simulink model "observerModel_GVS"  (R2024a)
settings: Solver=ode15s  StartTime=0.0  StopTime=duration  MaxStep=0.02  RelTol=0.02  AbsTol=0.02  EnableMultiTasking=on
values from neighbouring files (symbols this model uses):
  delta_t = time(2) - time (1)    [Observer_Analysis.m]
  f_oto = 2    [Observer_Analysis.m]
  f_scc = 2    [Observer_Analysis.m]
  GG0 = [0 0 -hypo]'    [Observer_Analysis.m]
  IrregDepol = tf(num,den)    [Observer_Analysis.m]
  IrregHyperpol = tf(num,den)    [Observer_Analysis.m]
  IrregSCC2Physical = inv(IrregSCCnf)    [Observer_Analysis.m]
  kaa = -4*[1 1 1]'    [Observer_Analysis.m]
  kfg = 4*[1 1 1]'    [Observer_Analysis.m]
  kfw = 8*[1 1 1]'    [Observer_Analysis.m]
  KGVS = s2(1)*pi/180    [Observer_Analysis.m]
  KLeft = 1-KRight    (= 0.5)    [Observer_Analysis.m]
  KReg = s2(2)    [Observer_Analysis.m]
  KRight = 0.5    [Observer_Analysis.m]
  kwg = 1*[1 1 1]'    [Observer_Analysis.m]
  kww = 8*[1 1 1]'    [Observer_Analysis.m]
  oto_a = 60*[1 1 1]'    [Observer_Analysis.m]
  oto_Ka = 1.3*[1 1 1]'    [Observer_Analysis.m]
  Q0 = [cos(E_angle/2) E(1)*sin(E_angle/2) E(2)*sin(E_angle/2) E(3)*sin(E_angle/2)]'    [Observer_Analysis.m]
  RegDepol = tf(num,den)    [Observer_Analysis.m]
  RegHyperpol = tf(num,den)    [Observer_Analysis.m]
  RegSCC2Physical = inv(RegSCCnf)    [Observer_Analysis.m]
  tau_a = tau_a_value*[1 1 1]'    [Observer_Analysis.m]
  tau_scc = tau_scc_value*[1 1 1]'    [Observer_Analysis.m]
(part 1 of 2)
settings Model: Creator=Newman  LastModifiedBy=caroa
settings SolverCC: AutoScaleAbsTol=off  AlgebraicLoopSolver=TrustRegion
settings DataIOCC: SaveFormat=Array  SignalLoggingSaveFormat=ModelDataLogs  SaveOutput=off  SaveTime=off  ReturnWorkspaceOutputs=off
settings OptimizationCC: ReuseModelBlockBuffer=off  ExpressionDepthLimit=2147483647  InitFltsAndDblsToZero=on  LifeSpan=inf
settings DebuggingCC: SaveWithParameterizedLinksMsg=none  UnderspecifiedInitializationDetection=Classic  MergeDetectMultiDrivingBlocksExec=none  SolverPrmCheckMsg=warning  FcnCallInpInsideContextMsg=warning  UnconnectedInputMsg=warning  UnconnectedOutputMsg=warning  UnconnectedLineMsg=warning  StateNameClashWarn=warning  SFUnexpectedBacktrackingDiag=warning  SFNoUnconditionalDefaultTransitionDiag=warning  SFExecutionAtInitializationDiag=none  ArithmeticOperatorsInVariantConditions=warning
settings HardwareCC: ProdBitPerPointer=32  ProdBitPerSizeT=32  ProdBitPerPtrDiffT=32  ProdLargestAtomicFloat=None  ProdIntDivRoundTo=Undefined  ProdEndianess=Unspecified  ProdWordSize=32  ProdHWDeviceType=32-bit Generic
settings ModelReferenceCC: EnableRefExpFcnMdlSchedulingChecks=on  PropagateSignalLabelsOutOfModel=off
settings SFSimCC: SimUseLocalCustomCode=off  CustomCodeUndefinedFunction=UseInterfaceOnly
settings RTWCC: RTWUseLocalCustomCode=off  GPUComputeCapability=3.5  DLArmComputeVersion=19.05
settings CodeAppCC: StateflowObjectComments=on
settings GRTTargetCC: TargetFcnLib=ansi_tfl_tmw.mat  TargetLangStandard=C89/C90 (ANSI)  CombineOutputUpdateFcns=off  GRTInterface=on
settings ConfigComp: CovMetricSettings=dw  CovSaveCumulativeToWorkspaceVar=on  CovSaveSingleToWorkspaceVar=on  CovExternalEMLEnable=off

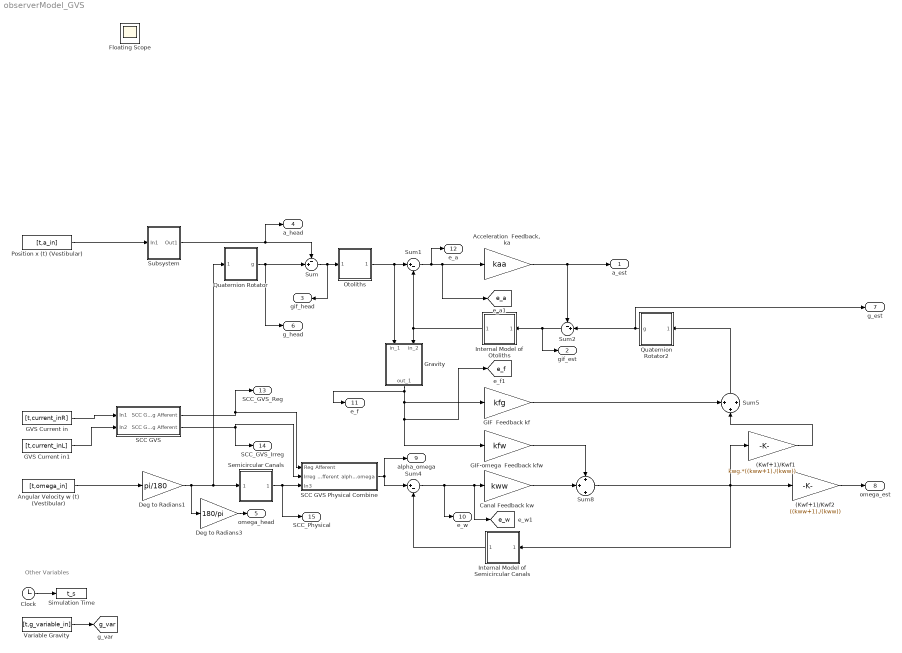
== system observerModel_GVS ==
  note: Other Variables
  (Kwf+1)/Kwf1 : Gain  Gain=kwg.*((kww+1)./(kww))  SaturateOnIntegerOverflow=on  OutDataTypeStr=Inherit: Same as input  ParamDataTypeStr=Inherit: Same as input
  (Kwf+1)/Kwf2 : Gain  Gain=((kww+1)./(kww))  SaturateOnIntegerOverflow=on  OutDataTypeStr=Inherit: Same as input  ParamDataTypeStr=Inherit: Same as input
  "Acceleration  Feedback, ka" : Gain  Gain=kaa  SaturateOnIntegerOverflow=on  OutDataTypeStr=Inherit: Same as input  ParamDataTypeStr=Inherit: Same as input
  Angular Velocity w (t) (Vestibular) : FromWorkspace  VariableName=[t,omega_in]  ZeroCross=off
  Canal Feedback kw : Gain  Gain=kww  SaturateOnIntegerOverflow=on  OutDataTypeStr=Inherit: Same as input  ParamDataTypeStr=Inherit: Same as input
  Clock : Clock
  Deg to Radians1 : Gain  Gain=pi/180  SaturateOnIntegerOverflow=on  OutDataTypeStr=Inherit: Same as input  ParamDataTypeStr=Inherit: Same as input
  Deg to Radians3 : Gain  Gain=180/pi  SaturateOnIntegerOverflow=on  OutDataTypeStr=Inherit: Same as input  ParamDataTypeStr=Inherit: Same as input
  GIF  Feedback kf : Gain  Gain=kfg  SaturateOnIntegerOverflow=on  OutDataTypeStr=Inherit: Same as input  ParamDataTypeStr=Inherit: Same as input
  GIF-omega  Feedback kfw : Gain  Gain=kfw  SaturateOnIntegerOverflow=on  OutDataTypeStr=Inherit: Same as input  ParamDataTypeStr=Inherit: Same as input
  GVS Current in : FromWorkspace  VariableName=[t,current_inR]  ZeroCross=off
  GVS Current in1 : FromWorkspace  VariableName=[t,current_inL]  ZeroCross=off
  Gravity : Subsystem
  Internal Model of Otoliths : Subsystem
      mask Display: fprintf('<OTO>')
  Internal Model of Semicircular Canals : Subsystem
      mask Display: fprintf('<SCC>')
  Otoliths : Subsystem
      mask Display: fprintf('OTO')
  Position x (t) (Vestibular) : FromWorkspace  VariableName=[t,a_in]  ZeroCross=off
  Quaternion Rotator : Subsystem
      mask Display: fprintf('G(w)')
  Quaternion Rotator2 : Subsystem
      mask Display: fprintf('Gest(w)')
  "SCC GVS " : Subsystem
  SCC GVS Physical Combine : Subsystem
  Semicircular Canals : Subsystem
      mask Display: fprintf('SCC')
  Simulation Time : ToWorkspace  VariableName=t_s
      settings: MaxDataPoints=100000
  Subsystem : Subsystem
      mask Display: fprintf('TH(w)')
  Sum : Sum  Inputs=-+|
  Sum1 : Sum  Inputs=|+-
  Sum2 : Sum  Inputs=-+|
  Sum4 : Sum  Inputs=|+-
  Sum5 : Sum  Inputs=+|+|+
  Sum8 : Sum  Inputs=+|+|+
  Variable Gravity : FromWorkspace  VariableName=[t,g_variable_in]  ZeroCross=off
  a_est : Outport
  gif_est : Outport  Port=2
  gif_head : Outport  Port=3
  a_head : Outport  Port=4
  omega_head : Outport  Port=5
  g_head : Outport  Port=6
  g_est : Outport  Port=7
  omega_est : Outport  Port=8
  alpha_omega : Outport  Port=9
  e_w : Outport  Port=10
  e_f : Outport  Port=11
  e_a : Outport  Port=12
  SCC_GVS_Reg : Outport  Port=13
  SCC_GVS_Irreg : Outport  Port=14
  SCC_Physical : Outport  Port=15
  Floating Scope : Scope
  tag scope: e_a=global, e_f=global, e_w=global, g_var=global
  wires:
  Clock/1 -> Simulation Time/1
  Quaternion Rotator/1(g) -> Sum/2, g_head/1
  Position x (t) (Vestibular)/1 -> Subsystem/1(In1)
  Sum/1 -> gif_head/1, Otoliths/1(Inport)
  Sum1/1 -> [e_a], "Acceleration  Feedback, ka"/1, e_a/1
  Otoliths/1(Outport) -> Sum1/1, Gravity/1(in_1)
  Sum2/1 -> gif_est/1, Internal Model of Otoliths/1(Inport)
  "Acceleration  Feedback, ka"/1 -> Sum2/1, a_est/1
  Gravity/1(out_1) -> GIF-omega  Feedback kfw/1, [e_f], GIF  Feedback kf/1, e_f/1
  GIF  Feedback kf/1 -> Sum5/1
  Sum5/1 -> Quaternion Rotator2/1(omega_rad_est)
  Sum4/1 -> [e_w], Canal Feedback kw/1, e_w/1
  GIF-omega  Feedback kfw/1 -> Sum8/1
  Canal Feedback kw/1 -> Sum8/2
  Internal Model of Semicircular Canals/1(Outport) -> Sum4/2
  Internal Model of Otoliths/1(Outport) -> Gravity/2(in_2), Sum1/2
  Sum8/1 -> (Kwf+1)/Kwf2/1, (Kwf+1)/Kwf1/1, Internal Model of Semicircular Canals/1(Inport)
  Quaternion Rotator2/1(g) -> g_est/1, Sum2/2
  Angular Velocity w (t) (Vestibular)/1 -> Deg to Radians1/1
  Deg to Radians3/1 -> omega_head/1
  Variable Gravity/1 -> [g_var]
  Deg to Radians1/1 -> Quaternion Rotator/1(omega_rad), Semicircular Canals/1(Inport), Deg to Radians3/1
  Subsystem/1(Out1) -> Sum/1, a_head/1
  (Kwf+1)/Kwf2/1 -> omega_est/1
  (Kwf+1)/Kwf1/1 -> Sum5/2
  GVS Current in/1 -> "SCC GVS "/1(In1)
  SCC GVS Physical Combine/1(alpha_omega) -> alpha_omega/1, Sum4/1
  "SCC GVS "/2(SCC GVS Irreg Afferent) -> SCC GVS Physical Combine/2(Irreg Afferent), SCC_GVS_Irreg/1
  "SCC GVS "/1(SCC GVS Reg Afferent) -> SCC_GVS_Reg/1, SCC GVS Physical Combine/1(Reg Afferent)
  Semicircular Canals/1(Outport) -> SCC_Physical/1, SCC GVS Physical Combine/3(In3)
  GVS Current in1/1 -> "SCC GVS "/2(In2)

== system observerModel_GVS/Gravity ==
  in_1 : Inport
  in_2 : Inport  Port=2
  Cross Product : Subsystem  mask(Nick's Library){}
      mask help: Cross Product
      mask Help: Cross Product
      mask Display: disp('--> -->\nu x v')
  Dot Product : DotProduct  OutDataTypeStr=Inherit: Inherit via internal rule
  Normalize : Subsystem
      mask Display: disp('->\nu\n__\n->\n|u|')
  Normalize1 : Subsystem
      mask Display: disp('->\nu\n__\n->\n|u|')
  Normalize2 : Subsystem
      mask Display: disp('->\nu\n__\n->\n|u|')
  Product : Product  InputSameDT=on  RndMeth=Zero  SaturateOnIntegerOverflow=on  OutDataTypeStr=Inherit: Same as first input
  Trigonometric Function : Trigonometry  Operator=acos
  out_1 : Outport  InitialOutput=0
  wires:
  Trigonometric Function/1 -> Product/2
  Product/1 -> out_1/1
  Normalize1/1(out_1) -> Dot Product/1
  Normalize/1(out_1) -> Dot Product/2
  in_1/1 -> Normalize1/1(in_1), Cross Product/1(in_1)
  Normalize2/1(out_1) -> Product/1
  Dot Product/1 -> Trigonometric Function/1
  Cross Product/1(out_1) -> Normalize2/1(in_1)
  in_2/1 -> Normalize/1(in_1), Cross Product/2(in_2)

== system observerModel_GVS/Internal Model of Otoliths ==
  note: Z otolith
  note: Y otolith
  note: X otolith
  Inport : Inport
  Demux : Demux  Outputs=3
      settings: DisplayOption=none
  Mux : Mux  Inputs=3
  Otolith : Subsystem
  Otolith1 : Subsystem
  Otolith2 : Subsystem
  Outport : Outport  InitialOutput=0
  wires:
  Otolith2/1(out_1) -> Mux/3
  Otolith/1(out_1) -> Mux/1
  Otolith1/1(out_1) -> Mux/2
  Demux/3 -> Otolith2/1(in_1)
  Demux/1 -> Otolith/1(in_1)
  Demux/2 -> Otolith1/1(in_1)
  Inport/1 -> Demux/1
  Mux/1 -> Outport/1

== system observerModel_GVS/Internal Model of Semicircular Canals ==
  note: Z canal
  note: Y canal
  note: X canal
  Inport : Inport
  Demux : Demux  Outputs=3
      settings: DisplayOption=none
  Mux : Mux  Inputs=3
  Zero-Pole : ZeroPole  Zeros=[0]  Poles=[-1/tau_scc(1);-2*pi*f_scc]  Gain=[(2*pi*f_scc)]
  Zero-Pole1 : ZeroPole  Zeros=[0]  Poles=[-1/tau_scc(2);-2*pi*f_scc]  Gain=[(2*pi*f_scc)]
  Zero-Pole2 : ZeroPole  Zeros=[0]  Poles=[-1/tau_scc(3);-2*pi*f_scc]  Gain=[(2*pi*f_scc)]
  Outport : Outport  InitialOutput=0
  wires:
  Inport/1 -> Demux/1
  Demux/3 -> Zero-Pole2/1
  Demux/1 -> Zero-Pole/1
  Demux/2 -> Zero-Pole1/1
  Zero-Pole2/1 -> Mux/3
  Zero-Pole1/1 -> Mux/2
  Zero-Pole/1 -> Mux/1
  Mux/1 -> Outport/1

== system observerModel_GVS/Otoliths ==
  Inport : Inport
  Demux : Demux  Outputs=3
      settings: DisplayOption=none
  Mux : Mux  Inputs=3
  X Graviceptor : Subsystem
  Y Graviceptor : Subsystem
  Z Graviceptor : Subsystem
  Outport : Outport  InitialOutput=0
  wires:
  Z Graviceptor/1(out_1) -> Mux/3
  X Graviceptor/1(out_1) -> Mux/1
  Y Graviceptor/1(out_1) -> Mux/2
  Demux/3 -> Z Graviceptor/1(in_1)
  Demux/1 -> X Graviceptor/1(in_1)
  Demux/2 -> Y Graviceptor/1(in_1)
  Inport/1 -> Demux/1
  Mux/1 -> Outport/1

== system observerModel_GVS/Quaternion Rotator ==
  omega_rad : Inport
  Head to Limbic Angular Velocity Transform : Subsystem
  Quaternion Integrator : Subsystem
  Quaternion to Direction Cosine : Subsystem
  Quaternion to Euler Angles : Subsystem
  Rotation : Subsystem
  SVV : ToWorkspace  VariableName=SVV  SampleTime=-1
  Tilt : ToWorkspace  VariableName=tilt  SampleTime=-1
  Tilt & SVV : Subsystem
  To Workspace : ToWorkspace  VariableName=azimuth_head  SampleTime=-1
  To Workspace2 : ToWorkspace  VariableName=euler_head  SampleTime=-1
  g : Outport
  tag scope: D_Cos=global, R_head=global
  wires:
  Quaternion Integrator/1(q) -> Quaternion to Direction Cosine/1(q), Quaternion to Euler Angles/1(q)
  Quaternion to Direction Cosine/1(D_Cos) -> Rotation/1(D_Cos), Head to Limbic Angular Velocity Transform/2(D_Cos), [D_Cos]
  omega_rad/1 -> Quaternion Integrator/1(omega_head), Rotation/2(omega_rad), Head to Limbic Angular Velocity Transform/1(omega_head)
  Rotation/1(g) -> g/1, Tilt & SVV/1(g)
  Rotation/2(azimuth) -> To Workspace/1
  Head to Limbic Angular Velocity Transform/1(R_limbic) -> [R_head]
  Quaternion to Euler Angles/1(Euler) -> To Workspace2/1
  Tilt & SVV/1(Tilt) -> Tilt/1
  Tilt & SVV/2(SVV) -> SVV/1

== system observerModel_GVS/Quaternion Rotator2 ==
  omega_rad_est : Inport
  Head to Limbic Angular Velocity Transform Rotation Matrix : Subsystem
  Quaternion Integrator : Subsystem
  Quaternion to Direction Cosine : Subsystem
  Quaternion to Euler Angles : Subsystem
  Rotation : Subsystem
  SVV Est : ToWorkspace  VariableName=SVV_est  SampleTime=-1
  Tilt & SVV : Subsystem
  Tilt Est : ToWorkspace  VariableName=tilt_est  SampleTime=-1
  To Workspace : ToWorkspace  VariableName=azimuth_est  SampleTime=-1
  To Workspace2 : ToWorkspace  VariableName=euler_est  SampleTime=-1
  g : Outport
  tag scope: D_Cos_est=global, R_est=global
  wires:
  Quaternion Integrator/1(q) -> Quaternion to Direction Cosine/1(q), Quaternion to Euler Angles/1(q)
  Quaternion to Direction Cosine/1(D_Cos) -> Rotation/1(D_Cos), [D_Cos_est], Head to Limbic Angular Velocity Transform Rotation Matrix/2(D_Cos)
  omega_rad_est/1 -> Quaternion Integrator/1(omega_rad_est), Rotation/2(omega_rad), Head to Limbic Angular Velocity Transform Rotation Matrix/1(omega_est)
  Rotation/1(g) -> g/1, Tilt & SVV/1(g)
  Rotation/2(azimuth) -> To Workspace/1
  Head to Limbic Angular Velocity Transform Rotation Matrix/1(R_limbic_est) -> [R_est]
  Quaternion to Euler Angles/1(Euler) -> To Workspace2/1
  Tilt & SVV/1(Tilt) -> Tilt Est/1
  Tilt & SVV/2(SVV) -> SVV Est/1

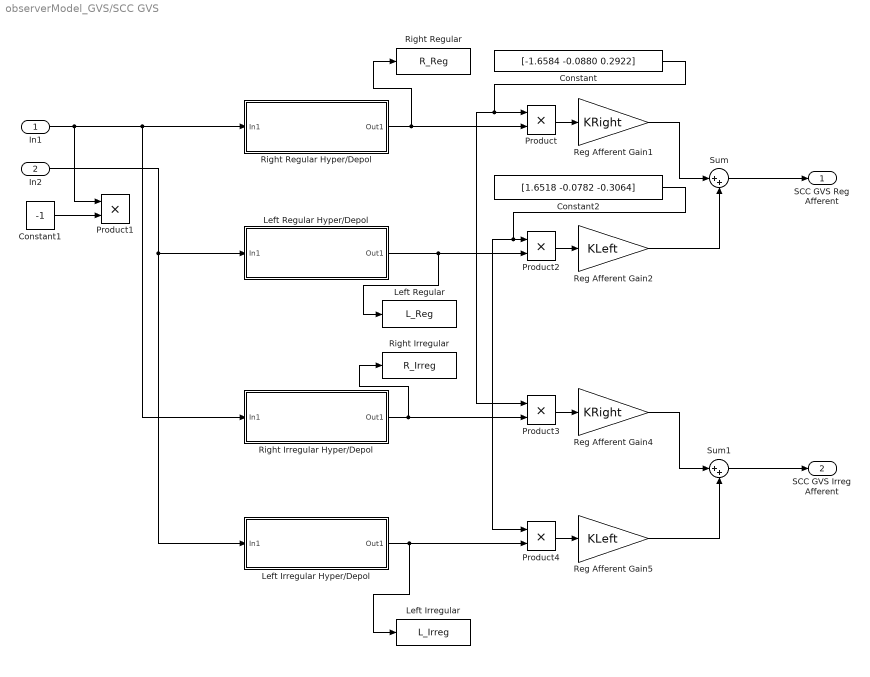
== system observerModel_GVS/SCC GVS  ==
  In1 : Inport
  In2 : Inport  Port=2
  Constant : Constant  Value=[-1.6584 -0.0880 0.2922]
  Constant1 : Constant  Value=-1
  Constant2 : Constant  Value=[1.6518 -0.0782 -0.3064]
  Left Irregular : ToWorkspace  VariableName=L_Irreg  SampleTime=-1
  "Left Irregular Hyper/Depol " : Subsystem
  Left Regular : ToWorkspace  VariableName=L_Reg  SampleTime=-1
  Left Regular Hyper/Depol : Subsystem
  Product{,1..4} (5 alike) : Product
  Reg Afferent Gain1 : Gain  Gain=KRight  SaturateOnIntegerOverflow=on  OutDataTypeStr=Inherit: Same as input  ParamDataTypeStr=Inherit: Same as input
  Reg Afferent Gain2 : Gain  Gain=KLeft  SaturateOnIntegerOverflow=on  OutDataTypeStr=Inherit: Same as input  ParamDataTypeStr=Inherit: Same as input
  Reg Afferent Gain4 : Gain  Gain=KRight  SaturateOnIntegerOverflow=on  OutDataTypeStr=Inherit: Same as input  ParamDataTypeStr=Inherit: Same as input
  Reg Afferent Gain5 : Gain  Gain=KLeft  SaturateOnIntegerOverflow=on  OutDataTypeStr=Inherit: Same as input  ParamDataTypeStr=Inherit: Same as input
  Right Irregular : ToWorkspace  VariableName=R_Irreg  SampleTime=-1
  "Right Irregular Hyper/Depol " : Subsystem
  Right Regular : ToWorkspace  VariableName=R_Reg  SampleTime=-1
  "Right Regular Hyper/Depol " : Subsystem
  Sum : Sum  Inputs=|++
  Sum1 : Sum  Inputs=|++
  SCC GVS Reg Afferent : Outport
  SCC GVS Irreg Afferent : Outport  Port=2
  wires:
  In1/1 -> "Right Regular Hyper/Depol "/1(In1), "Right Irregular Hyper/Depol "/1(In1), Product1/1
  Constant1/1 -> Product1/2
  In2/1 -> Left Regular Hyper/Depol/1(In1), "Left Irregular Hyper/Depol "/1(In1)
  Left Regular Hyper/Depol/1(Out1) -> Left Regular/1, Product2/2
  "Right Regular Hyper/Depol "/1(Out1) -> Right Regular/1, Product/2
  Constant/1 -> Product3/1, Product/1
  Constant2/1 -> Product4/1, Product2/1
  Product/1 -> Reg Afferent Gain1/1
  Product2/1 -> Reg Afferent Gain2/1
  Reg Afferent Gain1/1 -> Sum/1
  Reg Afferent Gain2/1 -> Sum/2
  Product3/1 -> Reg Afferent Gain4/1
  Reg Afferent Gain5/1 -> Sum1/2
  Reg Afferent Gain4/1 -> Sum1/1
  Product4/1 -> Reg Afferent Gain5/1
  "Left Irregular Hyper/Depol "/1(Out1) -> Left Irregular/1, Product4/2
  "Right Irregular Hyper/Depol "/1(Out1) -> Product3/2, Right Irregular/1
  Sum/1 -> SCC GVS Reg Afferent/1
  Sum1/1 -> SCC GVS Irreg Afferent/1

== system observerModel_GVS/SCC GVS Physical Combine ==
  Reg Afferent : Inport
  Irreg Afferent : Inport  Port=2
  In3 : Inport  Port=3
  Canal GVS Gain : Gain  Gain=KGVS  SaturateOnIntegerOverflow=on  OutDataTypeStr=Inherit: Same as input  ParamDataTypeStr=Inherit: Same as input
  Canal GVS Gain1 : Gain  Gain=KGVS  SaturateOnIntegerOverflow=on  OutDataTypeStr=Inherit: Same as input  ParamDataTypeStr=Inherit: Same as input
  Reg Afferent Gain : Gain  Gain=KReg  SaturateOnIntegerOverflow=on  OutDataTypeStr=Inherit: Same as input  ParamDataTypeStr=Inherit: Same as input
  Reg Afferent Gain3 : Gain  Gain=1-KReg  SaturateOnIntegerOverflow=on  OutDataTypeStr=Inherit: Same as input  ParamDataTypeStr=Inherit: Same as input
  Sum12 : Sum  Inputs=|++
  Sum13 : Sum  Inputs=|++
  Sum14 : Sum  Inputs=|++
  alpha_omega : Outport
  wires:
  Sum14/1 -> Reg Afferent Gain/1
  Sum12/1 -> Reg Afferent Gain3/1
  In3/1 -> Sum14/2, Sum12/2
  Irreg Afferent/1 -> Canal GVS Gain1/1
  Reg Afferent/1 -> Canal GVS Gain/1
  Sum13/1 -> alpha_omega/1
  Reg Afferent Gain/1 -> Sum13/1
  Reg Afferent Gain3/1 -> Sum13/2
  Canal GVS Gain/1 -> Sum14/1
  Canal GVS Gain1/1 -> Sum12/1

== system observerModel_GVS/Semicircular Canals ==
  note: Z canal
  note: Y canal
  note: X canal
  Inport : Inport
  Demux : Demux  Outputs=3
      settings: DisplayOption=none
  Mux : Mux  Inputs=3
  Zero-Pole : ZeroPole  Zeros=[0;0]  Poles=[-1/tau_scc(1);-1/tau_a(1);-2*pi*f_scc]  Gain=[(2*pi*f_scc)]
  Zero-Pole1 : ZeroPole  Zeros=[0;0]  Poles=[-1/tau_scc(2);-1/tau_a(2);-2*pi*f_scc]  Gain=[(2*pi*f_scc)]
  Zero-Pole2 : ZeroPole  Zeros=[0;0]  Poles=[-1/tau_scc(3);-1/tau_a(3);-2*pi*f_scc]  Gain=[(2*pi*f_scc)]
  Outport : Outport  InitialOutput=0
  wires:
  Demux/3 -> Zero-Pole2/1
  Demux/1 -> Zero-Pole/1
  Demux/2 -> Zero-Pole1/1
  Zero-Pole2/1 -> Mux/3
  Zero-Pole1/1 -> Mux/2
  Zero-Pole/1 -> Mux/1
  Inport/1 -> Demux/1
  Mux/1 -> Outport/1

== system observerModel_GVS/Subsystem ==
  In1 : Inport
  Deg to Radians4 : Gain  Gain=1/9.80665  SaturateOnIntegerOverflow=on  OutDataTypeStr=Inherit: Same as input  ParamDataTypeStr=Inherit: Same as input
  Matrix Multiplication : Subsystem
  Out1 : Outport
  wires:
  [D_Cos] -> Matrix Multiplication/1(D_Cos)
  In1/1 -> Deg to Radians4/1
  Matrix Multiplication/1(a_head) -> Out1/1
  Deg to Radians4/1 -> Matrix Multiplication/2(a_world)

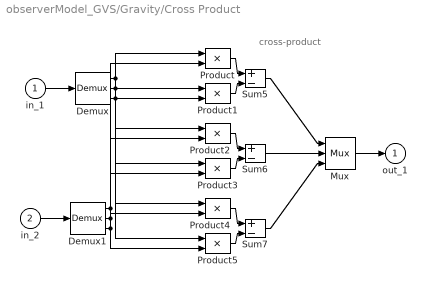
== system observerModel_GVS/Gravity/Cross Product ==
  note: cross-product
  in_1 : Inport
  in_2 : Inport  Port=2
  Demux : Demux  Outputs=3
      settings: DisplayOption=none
  Demux1 : Demux  Outputs=3
      settings: DisplayOption=none
  Mux : Mux  Inputs=3
  Product{,1..5} (6 alike) : Product  InputSameDT=on  RndMeth=Zero  SaturateOnIntegerOverflow=on  OutDataTypeStr=Inherit: Same as first input
  Sum5 : Sum  Inputs=+-  InputSameDT=on  SaturateOnIntegerOverflow=on  OutDataTypeStr=Inherit: Same as first input
  Sum6 : Sum  Inputs=+-  InputSameDT=on  SaturateOnIntegerOverflow=on  OutDataTypeStr=Inherit: Same as first input
  Sum7 : Sum  Inputs=+-  InputSameDT=on  SaturateOnIntegerOverflow=on  OutDataTypeStr=Inherit: Same as first input
  out_1 : Outport  InitialOutput=0
  wires:
  in_2/1 -> Demux1/1
  Mux/1 -> out_1/1
  in_1/1 -> Demux/1
  Product/1 -> Sum5/1
  Product1/1 -> Sum5/2
  Product2/1 -> Sum6/1
  Product3/1 -> Sum6/2
  Product4/1 -> Sum7/1
  Product5/1 -> Sum7/2
  Sum5/1 -> Mux/1
  Sum6/1 -> Mux/2
  Sum7/1 -> Mux/3
  Demux/3 -> Product1/1, Product2/1
  Demux1/3 -> Product/2, Product3/2
  Demux/1 -> Product3/1, Product4/1
  Demux1/2 -> Product1/2, Product4/2
  Demux/2 -> Product/1, Product5/1
  Demux1/1 -> Product2/2, Product5/2

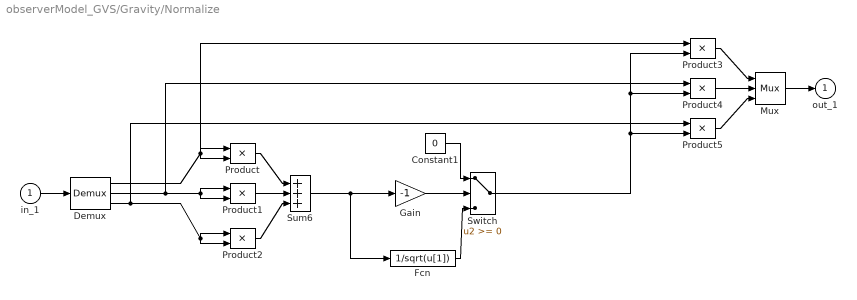
== system observerModel_GVS/Gravity/Normalize ==
  in_1 : Inport
  Constant1 : Constant  Value=0
  Demux : Demux  Outputs=3
      settings: DisplayOption=none
  Fcn : Fcn  Expr=1/sqrt(u[1])
  Gain : Gain  Gain=-1  SaturateOnIntegerOverflow=on  OutDataTypeStr=Inherit: Same as input  ParamDataTypeStr=Inherit: Same as input
  Mux : Mux  Inputs=3
  Product{,1..5} (6 alike) : Product  InputSameDT=on  RndMeth=Zero  SaturateOnIntegerOverflow=on  OutDataTypeStr=Inherit: Same as first input
  Sum6 : Sum  Inputs=+++  InputSameDT=on  SaturateOnIntegerOverflow=on  OutDataTypeStr=Inherit: Same as first input
  Switch : Switch
  out_1 : Outport  InitialOutput=0
  wires:
  Sum6/1 -> Gain/1, Fcn/1
  Fcn/1 -> Switch/3
  Constant1/1 -> Switch/1
  Switch/1 -> Product5/2, Product3/2, Product4/2
  Product5/1 -> Mux/3
  Product3/1 -> Mux/1
  Product4/1 -> Mux/2
  Demux/2 -> Product4/1, Product1/1, Product1/2
  Demux/3 -> Product5/1, Product2/2, Product2/1
  Demux/1 -> Product/2, Product/1, Product3/1
  Product1/1 -> Sum6/2
  Product/1 -> Sum6/1
  Product2/1 -> Sum6/3
  Mux/1 -> out_1/1
  in_1/1 -> Demux/1
  Gain/1 -> Switch/2

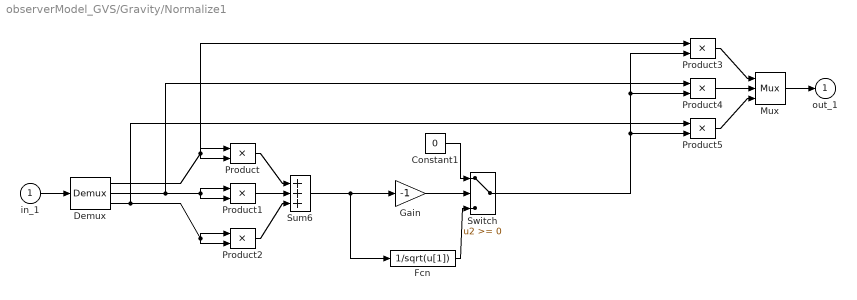
== system observerModel_GVS/Gravity/Normalize1 ==
  in_1 : Inport
  Constant1 : Constant  Value=0
  Demux : Demux  Outputs=3
      settings: DisplayOption=none
  Fcn : Fcn  Expr=1/sqrt(u[1])
  Gain : Gain  Gain=-1  SaturateOnIntegerOverflow=on  OutDataTypeStr=Inherit: Same as input  ParamDataTypeStr=Inherit: Same as input
  Mux : Mux  Inputs=3
  Product{,1..5} (6 alike) : Product  InputSameDT=on  RndMeth=Zero  SaturateOnIntegerOverflow=on  OutDataTypeStr=Inherit: Same as first input
  Sum6 : Sum  Inputs=+++  InputSameDT=on  SaturateOnIntegerOverflow=on  OutDataTypeStr=Inherit: Same as first input
  Switch : Switch
  out_1 : Outport  InitialOutput=0
  wires:
  Sum6/1 -> Gain/1, Fcn/1
  Fcn/1 -> Switch/3
  Constant1/1 -> Switch/1
  Switch/1 -> Product5/2, Product3/2, Product4/2
  Product5/1 -> Mux/3
  Product3/1 -> Mux/1
  Product4/1 -> Mux/2
  Demux/2 -> Product4/1, Product1/1, Product1/2
  Demux/3 -> Product5/1, Product2/2, Product2/1
  Demux/1 -> Product/2, Product/1, Product3/1
  Product1/1 -> Sum6/2
  Product/1 -> Sum6/1
  Product2/1 -> Sum6/3
  Mux/1 -> out_1/1
  in_1/1 -> Demux/1
  Gain/1 -> Switch/2

== system observerModel_GVS/Gravity/Normalize2 ==
  in_1 : Inport
  Constant1 : Constant  Value=inf
  Demux : Demux  Outputs=3
      settings: DisplayOption=none
  Fcn : Fcn  Expr=1/sqrt(u)
  Gain : Gain  Gain=-1  SaturateOnIntegerOverflow=on  OutDataTypeStr=Inherit: Same as input  ParamDataTypeStr=Inherit: Same as input
  Mux : Mux  Inputs=3
  Product{,1..5} (6 alike) : Product  InputSameDT=on  RndMeth=Zero  SaturateOnIntegerOverflow=on  OutDataTypeStr=Inherit: Same as first input
  Sum6 : Sum  Inputs=+++  InputSameDT=on  SaturateOnIntegerOverflow=on  OutDataTypeStr=Inherit: Same as first input
  Switch : Switch
  out_1 : Outport  InitialOutput=0
  wires:
  Sum6/1 -> Gain/1, Switch/3
  Constant1/1 -> Switch/1
  Product5/1 -> Mux/3
  Product3/1 -> Mux/1
  Product4/1 -> Mux/2
  Demux/2 -> Product4/1, Product1/1, Product1/2
  Demux/3 -> Product5/1, Product2/2, Product2/1
  Demux/1 -> Product/2, Product/1, Product3/1
  Product1/1 -> Sum6/2
  Product/1 -> Sum6/1
  Product2/1 -> Sum6/3
  Mux/1 -> out_1/1
  in_1/1 -> Demux/1
  Gain/1 -> Switch/2
  Switch/1 -> Fcn/1
  Fcn/1 -> Product5/2, Product3/2, Product4/2

== system observerModel_GVS/Internal Model of Otoliths/Otolith ==
  in_1 : Inport
  Transfer Fcn3 : TransferFcn  Denominator=[1/(2*pi*f_oto) 1]
  out_1 : Outport  InitialOutput=0
  wires:
  in_1/1 -> Transfer Fcn3/1
  Transfer Fcn3/1 -> out_1/1

== system observerModel_GVS/Internal Model of Otoliths/Otolith1 ==
  in_1 : Inport
  Transfer Fcn3 : TransferFcn  Denominator=[1/(2*pi*f_oto) 1]
  out_1 : Outport  InitialOutput=0
  wires:
  in_1/1 -> Transfer Fcn3/1
  Transfer Fcn3/1 -> out_1/1

== system observerModel_GVS/Internal Model of Otoliths/Otolith2 ==
  in_1 : Inport
  Transfer Fcn3 : TransferFcn  Denominator=[1/(2*pi*f_oto) 1]
  out_1 : Outport  InitialOutput=0
  wires:
  Transfer Fcn3/1 -> out_1/1
  in_1/1 -> Transfer Fcn3/1

== system observerModel_GVS/Otoliths/X Graviceptor ==
  in_1 : Inport
  Adaptation : TransferFcn  Numerator=[oto_Ka(1)*oto_a(1) 1]  Denominator=[oto_a(1) 1]
  Low Pass Filter : TransferFcn  Denominator=[1/(2*pi*f_oto) 1]
  New Otolith model : TransferFcn  Numerator=[333 33.3]  Denominator="[0.08  5.016 1]"
  Scope{,1..3} (4 alike) : Scope
  X Graviceptor : TransferFcn  Numerator=[oto_Ka(1)*oto_a(1) 1]  Denominator=[oto_a(1)*1/(2*pi*f_oto) (1/(2*pi*f_oto)+oto_a(1)) 1]
  out_1 : Outport  InitialOutput=0
  wires:
  in_1/1 -> Low Pass Filter/1, X Graviceptor/1, Adaptation/1, New Otolith model/1
  Low Pass Filter/1 -> out_1/1, Scope2/1
  X Graviceptor/1 -> Scope/1
  Adaptation/1 -> Scope1/1
  New Otolith model/1 -> Scope3/1

== system observerModel_GVS/Otoliths/Y Graviceptor ==
  in_1 : Inport
  Adaptation : TransferFcn  Numerator=[oto_Ka(2)*oto_a(2) 1]  Denominator=[oto_a(2) 1]
  Low Pass Filter : TransferFcn  Denominator=[1/(2*pi*f_oto) 1]
  New Otolith model : TransferFcn  Numerator=[333 33.3]  Denominator="[0.08  5.016 1]"
  Scope{,1..3} (4 alike) : Scope
  X Graviceptor : TransferFcn  Numerator=[oto_Ka(2)*oto_a(2) 1]  Denominator=[oto_a(2)*1/(2*pi*f_oto) (1/(2*pi*f_oto)+oto_a(2)) 1]
  out_1 : Outport  InitialOutput=0
  wires:
  in_1/1 -> Low Pass Filter/1, X Graviceptor/1, Adaptation/1, New Otolith model/1
  Low Pass Filter/1 -> out_1/1, Scope2/1
  X Graviceptor/1 -> Scope/1
  Adaptation/1 -> Scope1/1
  New Otolith model/1 -> Scope3/1

== system observerModel_GVS/Otoliths/Z Graviceptor ==
  in_1 : Inport
  Adaptation : TransferFcn  Numerator=[oto_Ka(3)*oto_a(3) 1]  Denominator=[oto_a(3) 1]
  Low Pass Filter : TransferFcn  Denominator=[1/(2*pi*f_oto) 1]
  New Otolith model : TransferFcn  Numerator=[333 33.3]  Denominator="[0.08  5.016 1]"
  Scope{,1..3} (4 alike) : Scope
  X Graviceptor : TransferFcn  Numerator=[oto_Ka(3)*oto_a(3) 1]  Denominator=[oto_a(3)*1/(2*pi*f_oto) (1/(2*pi*f_oto)+oto_a(3)) 1]
  out_1 : Outport  InitialOutput=0
  wires:
  Low Pass Filter/1 -> out_1/1, Scope2/1
  X Graviceptor/1 -> Scope/1
  Adaptation/1 -> Scope1/1
  New Otolith model/1 -> Scope3/1
  in_1/1 -> Low Pass Filter/1, X Graviceptor/1, Adaptation/1, New Otolith model/1

== system observerModel_GVS/Quaternion Rotator/Head to Limbic Angular Velocity Transform ==
  omega_head : Inport
  D_Cos : Inport  Port=2
  Gain : Gain  Gain=-1
  Product1 : Product  Multiplication=Matrix(*)  RndMeth=Zero
  Quaternion Integrator1 : Subsystem
  Quaternion to Direction Cosine1 : Subsystem
  Transform Axes : Subsystem
  Transpose : Math  Operator=transpose  SignedPower=on
  R_limbic : Outport
  wires:
  Quaternion Integrator1/1(q) -> Quaternion to Direction Cosine1/1(q)
  Quaternion to Direction Cosine1/1(D_Cos) -> R_limbic/1
  omega_head/1 -> Product1/2
  Transpose/1 -> Product1/1
  D_Cos/1 -> Transpose/1
  Product1/1 -> Transform Axes/1(limbic_cord)
  Transform Axes/1(VR_cord) -> Gain/1
  Gain/1 -> Quaternion Integrator1/1(omega_limbic)

== system observerModel_GVS/Quaternion Rotator/Quaternion Integrator ==
  omega_head : Inport
  Demux1 : Demux
  Gain : Gain  Gain=1/delta_t
  Mux1 : Mux
  delta_q : Subsystem
  q0 : Integrator  InitialCondition=Q0(1)
  q1 : Integrator  InitialCondition=Q0(2)
  q2 : Integrator  InitialCondition=Q0(3)
  q3 : Integrator  InitialCondition=Q0(4)
  q : Outport
  wires:
  Demux1/1 -> q0/1
  q0/1 -> Mux1/1
  Demux1/2 -> q1/1
  q1/1 -> Mux1/2
  Demux1/3 -> q2/1
  q2/1 -> Mux1/3
  Demux1/4 -> q3/1
  q3/1 -> Mux1/4
  Mux1/1 -> delta_q/2(q), q/1
  Gain/1 -> Demux1/1
  delta_q/1(delta_q) -> Gain/1
  omega_head/1 -> delta_q/1(omega)

== system observerModel_GVS/Quaternion Rotator/Quaternion to Direction Cosine ==
  note: A21
  q : Inport
  A1 : Subsystem
  A11 : Subsystem
  A12 : Subsystem
  A13 : Subsystem
  A22 : Subsystem
  A23 : Subsystem
  A31 : Subsystem
  A32 : Subsystem
  A33 : Subsystem
  Mux : Mux  Inputs=9
  Reshape (9) to [3x3] column-major : Reshape  OutputDimensionality=Customize  OutputDimensions=[3,3]
  D_Cos : Outport
  wires:
  A33/1(A33) -> Mux/9
  A32/1(A32) -> Mux/6
  A31/1(A31) -> Mux/3
  A23/1(A23) -> Mux/8
  A22/1(A22) -> Mux/5
  A13/1(A13) -> Mux/7
  A12/1(A12) -> Mux/4
  A11/1(A11) -> Mux/1
  q/1 -> A22/1(q), A1/1(q), A13/1(q), A12/1(q), A11/1(q), A23/1(q), A31/1(q), A32/1(q), A33/1(q)
  Reshape (9) to [3x3] column-major/1 -> D_Cos/1
  A1/1(A21) -> Mux/2
  Mux/1 -> Reshape (9) to [3x3] column-major/1

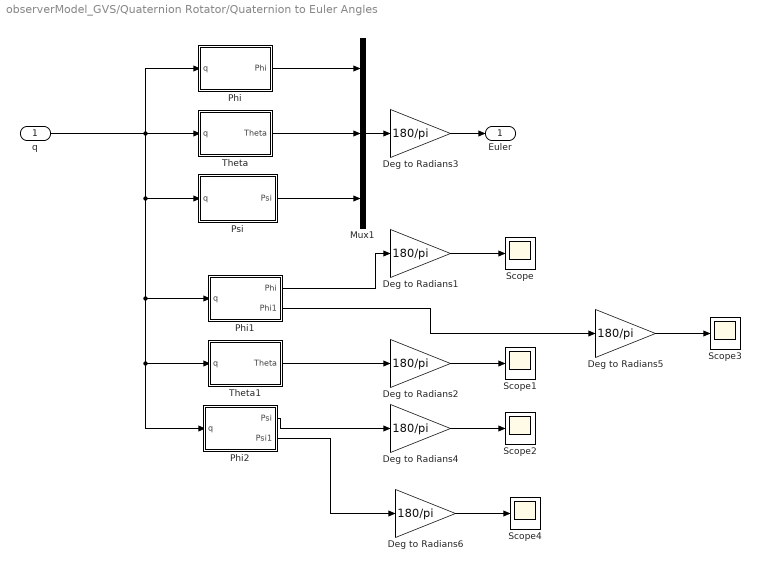
== system observerModel_GVS/Quaternion Rotator/Quaternion to Euler Angles ==
  q : Inport
  Deg to Radians{1..6} (6 alike) : Gain  Gain=180/pi  SaturateOnIntegerOverflow=on  OutDataTypeStr=Inherit: Same as input  ParamDataTypeStr=Inherit: Same as input
  Mux1 : Mux  Inputs=3
  Phi : Subsystem
  Phi1 : Subsystem
  Phi2 : Subsystem
  Psi : Subsystem
  Scope{,1..4} (5 alike) : Scope
  Theta : Subsystem
  Theta1 : Subsystem
  Euler : Outport
  wires:
  Phi/1(Phi) -> Mux1/1
  Psi/1(Psi) -> Mux1/3
  Theta/1(Theta) -> Mux1/2
  q/1 -> Theta/1(q), Phi/1(q), Psi/1(q), Phi1/1(q), Theta1/1(q), Phi2/1(q)
  Mux1/1 -> Deg to Radians3/1
  Deg to Radians3/1 -> Euler/1
  Deg to Radians1/1 -> Scope/1
  Deg to Radians2/1 -> Scope1/1
  Deg to Radians4/1 -> Scope2/1
  Phi1/1(Phi) -> Deg to Radians1/1
  Theta1/1(Theta) -> Deg to Radians2/1
  Phi2/1(Psi) -> Deg to Radians4/1
  Deg to Radians5/1 -> Scope3/1
  Phi1/2(Phi1) -> Deg to Radians5/1
  Deg to Radians6/1 -> Scope4/1
  Phi2/2(Psi1) -> Deg to Radians6/1

== system observerModel_GVS/Quaternion Rotator/Rotation ==
  D_Cos : Inport
  omega_rad : Inport  Port=2
  Azimuthal Integrator : Subsystem
  Ground Truth Gravity over time : FromWorkspace  VariableName=[t,G0]  ZeroCross=off
  Matrix Multiplication : Subsystem
  g : Outport
  azimuth : Outport  Port=2
  wires:
  D_Cos/1 -> Matrix Multiplication/1(D_Cos), Azimuthal Integrator/2(D_Cos)
  Matrix Multiplication/1(g) -> g/1, Azimuthal Integrator/1(g)
  omega_rad/1 -> Azimuthal Integrator/3(omega_rad)
  Azimuthal Integrator/1(azimuth) -> azimuth/1
  Ground Truth Gravity over time/1 -> Matrix Multiplication/2(G0)

== system observerModel_GVS/Quaternion Rotator/Tilt & SVV ==
  g : Inport
  SVV Calculator : Subsystem
  Tilt Calculator : Subsystem
  Tilt : Outport
  SVV : Outport  Port=2
  wires:
  g/1 -> SVV Calculator/1(g), Tilt Calculator/1(g)
  Tilt Calculator/1(Tilt) -> Tilt/1
  SVV Calculator/1(SVV) -> SVV/1

== system observerModel_GVS/Quaternion Rotator2/Head to Limbic Angular Velocity Transform Rotation Matrix ==
  omega_est : Inport
  D_Cos : Inport  Port=2
  Gain : Gain  Gain=-1
  Product1 : Product  Multiplication=Matrix(*)  RndMeth=Zero
  Quaternion Integrator1 : Subsystem
  Quaternion to Direction Cosine1 : Subsystem
  Transform Axes : Subsystem
  Transpose : Math  Operator=transpose  SignedPower=on
  R_limbic_est : Outport
  wires:
  Quaternion Integrator1/1(q) -> Quaternion to Direction Cosine1/1(q)
  Quaternion to Direction Cosine1/1(D_Cos) -> R_limbic_est/1
  omega_est/1 -> Product1/2
  Transpose/1 -> Product1/1
  D_Cos/1 -> Transpose/1
  Product1/1 -> Transform Axes/1(limbic_cord)
  Transform Axes/1(VR_cord) -> Gain/1
  Gain/1 -> Quaternion Integrator1/1(omega_limbic)

== system observerModel_GVS/Quaternion Rotator2/Quaternion Integrator ==
  omega_rad_est : Inport
  Demux1 : Demux
  Gain : Gain  Gain=1/delta_t
  Mux1 : Mux
  delta_q : Subsystem
  q0 : Integrator  InitialCondition=Q0(1)
  q1 : Integrator  InitialCondition=Q0(2)
  q2 : Integrator  InitialCondition=Q0(3)
  q3 : Integrator  InitialCondition=Q0(4)
  q : Outport
  wires:
  Demux1/1 -> q0/1
  q0/1 -> Mux1/1
  Demux1/2 -> q1/1
  q1/1 -> Mux1/2
  Demux1/3 -> q2/1
  q2/1 -> Mux1/3
  Demux1/4 -> q3/1
  q3/1 -> Mux1/4
  Mux1/1 -> delta_q/2(q), q/1
  Gain/1 -> Demux1/1
  delta_q/1(delta_q) -> Gain/1
  omega_rad_est/1 -> delta_q/1(omega)

== system observerModel_GVS/Quaternion Rotator2/Quaternion to Direction Cosine ==
  note: A21
  q : Inport
  A1 : Subsystem
  A11 : Subsystem
  A12 : Subsystem
  A13 : Subsystem
  A22 : Subsystem
  A23 : Subsystem
  A31 : Subsystem
  A32 : Subsystem
  A33 : Subsystem
  Mux : Mux  Inputs=9
  Reshape (9) to [3x3] column-major : Reshape  OutputDimensionality=Customize  OutputDimensions=[3,3]
  D_Cos : Outport
  wires:
  A33/1(A33) -> Mux/9
  A32/1(A32) -> Mux/6
  A31/1(A31) -> Mux/3
  A23/1(A23) -> Mux/8
  A22/1(A22) -> Mux/5
  A13/1(A13) -> Mux/7
  A12/1(A12) -> Mux/4
  A11/1(A11) -> Mux/1
  q/1 -> A22/1(q), A1/1(q), A13/1(q), A12/1(q), A11/1(q), A23/1(q), A31/1(q), A32/1(q), A33/1(q)
  Reshape (9) to [3x3] column-major/1 -> D_Cos/1
  A1/1(A21) -> Mux/2
  Mux/1 -> Reshape (9) to [3x3] column-major/1

== system observerModel_GVS/Quaternion Rotator2/Quaternion to Euler Angles ==
  q : Inport
  Deg to Radians3 : Gain  Gain=180/pi  SaturateOnIntegerOverflow=on  OutDataTypeStr=Inherit: Same as input  ParamDataTypeStr=Inherit: Same as input
  Mux1 : Mux  Inputs=3
  Phi : Subsystem
  Psi : Subsystem
  Theta : Subsystem
  Euler : Outport
  wires:
  Phi/1(Phi) -> Mux1/1
  Psi/1(Psi) -> Mux1/3
  Theta/1(Theta) -> Mux1/2
  q/1 -> Phi/1(q), Theta/1(q), Psi/1(q)
  Mux1/1 -> Deg to Radians3/1
  Deg to Radians3/1 -> Euler/1

== system observerModel_GVS/Quaternion Rotator2/Rotation ==
  D_Cos : Inport
  omega_rad : Inport  Port=2
  Azimuthal Integrator : Subsystem
  Hypo Gravity State : Constant  Value=GG0  VectorParams1D=off
  Matrix Multiplication : Subsystem
  g : Outport
  azimuth : Outport  Port=2
  wires:
  Hypo Gravity State/1 -> Matrix Multiplication/2(GG0)
  D_Cos/1 -> Matrix Multiplication/1(D_Cos), Azimuthal Integrator/2(D_Cos)
  Matrix Multiplication/1(g) -> g/1, Azimuthal Integrator/1(g)
  omega_rad/1 -> Azimuthal Integrator/3(omega_rad)
  Azimuthal Integrator/1(azimuth) -> azimuth/1

== system observerModel_GVS/Quaternion Rotator2/Tilt & SVV ==
  g : Inport
  SVV Calculator : Subsystem
  Tilt Calculator : Subsystem
  Tilt : Outport
  SVV : Outport  Port=2
  wires:
  g/1 -> Tilt Calculator/1(g), SVV Calculator/1(g)
  Tilt Calculator/1(Tilt) -> Tilt/1
  SVV Calculator/1(SVV) -> SVV/1

== system observerModel_GVS/SCC GVS /Left Irregular Hyper//Depol  ==
  In1 : Inport
  If : If
  If Action Subsystem : Subsystem  TreatAsAtomicUnit=on
  If Action Subsystem1 : Subsystem  TreatAsAtomicUnit=on
  Merge : Merge
  Out1 : Outport
  wires:
  In1/1 -> If Action Subsystem1/1(In1), If Action Subsystem/1(In1), If/1
  Merge/1 -> Out1/1
  If/1 -> If Action Subsystem/Action
  If Action Subsystem/1(Out1) -> Merge/1
  If Action Subsystem1/1(Out1) -> Merge/2
  If/2 -> If Action Subsystem1/Action

== system observerModel_GVS/SCC GVS /Left Regular Hyper//Depol ==
  In1 : Inport
  If : If
  If Action Subsystem : Subsystem  TreatAsAtomicUnit=on
  If Action Subsystem1 : Subsystem  TreatAsAtomicUnit=on
  Merge : Merge
  Out1 : Outport
  wires:
  In1/1 -> If Action Subsystem1/1(In1), If Action Subsystem/1(In1), If/1
  Merge/1 -> Out1/1
  If/1 -> If Action Subsystem/Action
  If Action Subsystem/1(Out1) -> Merge/1
  If Action Subsystem1/1(Out1) -> Merge/2
  If/2 -> If Action Subsystem1/Action

== system observerModel_GVS/SCC GVS /Right Irregular Hyper//Depol  ==
  In1 : Inport
  If : If
  If Action Subsystem : Subsystem  TreatAsAtomicUnit=on
  If Action Subsystem1 : Subsystem  TreatAsAtomicUnit=on
  Merge : Merge
  Out1 : Outport
  wires:
  In1/1 -> If Action Subsystem1/1(In1), If Action Subsystem/1(In1), If/1
  Merge/1 -> Out1/1
  If/1 -> If Action Subsystem/Action
  If Action Subsystem/1(Out1) -> Merge/1
  If Action Subsystem1/1(Out1) -> Merge/2
  If/2 -> If Action Subsystem1/Action

== system observerModel_GVS/SCC GVS /Right Regular Hyper//Depol  ==
  In1 : Inport
  If : If
  If Action Subsystem : Subsystem  TreatAsAtomicUnit=on
  If Action Subsystem1 : Subsystem  TreatAsAtomicUnit=on
  Merge : Merge
  Out1 : Outport
  wires:
  In1/1 -> If Action Subsystem1/1(In1), If Action Subsystem/1(In1), If/1
  Merge/1 -> Out1/1
  If/1 -> If Action Subsystem/Action
  If Action Subsystem/1(Out1) -> Merge/1
  If Action Subsystem1/1(Out1) -> Merge/2
  If/2 -> If Action Subsystem1/Action

== system observerModel_GVS/Subsystem/Matrix Multiplication ==
  D_Cos : Inport
  a_world : Inport  Port=2
  Demux : Demux  Outputs=3
      settings: DisplayOption=none
  Mux : Mux  Inputs=3
  Product : Product  Multiplication=Matrix(*)  RndMeth=Zero
  a_head : Outport
  wires:
  Product/1 -> Demux/1
  Demux/1 -> Mux/1
  Demux/2 -> Mux/2
  Demux/3 -> Mux/3
  D_Cos/1 -> Product/1
  Mux/1 -> a_head/1
  a_world/1 -> Product/2

== system observerModel_GVS/Quaternion Rotator/Head to Limbic Angular Velocity Transform/Quaternion Integrator1 ==
  omega_limbic : Inport
  Demux1 : Demux
  Gain : Gain  Gain=1/delta_t
  Mux1 : Mux
  delta_q : Subsystem
  q0 : Integrator  InitialCondition=Q0(1)
  q1 : Integrator  InitialCondition=Q0(3)
  q2 : Integrator  InitialCondition=Q0(4)
  q3 : Integrator  InitialCondition=Q0(2)
  q : Outport
  wires:
  Demux1/1 -> q0/1
  Demux1/2 -> q1/1
  Demux1/3 -> q2/1
  Demux1/4 -> q3/1
  Mux1/1 -> delta_q/2(q), q/1
  Gain/1 -> Demux1/1
  delta_q/1(delta_q) -> Gain/1
  omega_limbic/1 -> delta_q/1(omega)
  q0/1 -> Mux1/1
  q2/1 -> Mux1/3
  q3/1 -> Mux1/4
  q1/1 -> Mux1/2

== system observerModel_GVS/Quaternion Rotator/Head to Limbic Angular Velocity Transform/Quaternion to Direction Cosine1 ==
  note: A21
  q : Inport
  A1 : Subsystem
  A11 : Subsystem
  A12 : Subsystem
  A13 : Subsystem
  A22 : Subsystem
  A23 : Subsystem
  A31 : Subsystem
  A32 : Subsystem
  A33 : Subsystem
  Mux : Mux  Inputs=9
  Reshape (9) to [3x3] column-major : Reshape  OutputDimensionality=Customize  OutputDimensions=[3,3]
  D_Cos : Outport
  wires:
  A33/1(A33) -> Mux/9
  A32/1(A32) -> Mux/6
  A31/1(A31) -> Mux/3
  A23/1(A23) -> Mux/8
  A22/1(A22) -> Mux/5
  A13/1(A13) -> Mux/7
  A12/1(A12) -> Mux/4
  A11/1(A11) -> Mux/1
  q/1 -> A22/1(q), A1/1(q), A13/1(q), A12/1(q), A11/1(q), A23/1(q), A31/1(q), A32/1(q), A33/1(q)
  Reshape (9) to [3x3] column-major/1 -> D_Cos/1
  A1/1(A21) -> Mux/2
  Mux/1 -> Reshape (9) to [3x3] column-major/1

== system observerModel_GVS/Quaternion Rotator/Head to Limbic Angular Velocity Transform/Transform Axes ==
  limbic_cord : Inport
  Demux2 : Demux  Outputs=3
  Mux2 : Mux  Inputs=3
  VR_cord : Outport
  wires:
  limbic_cord/1 -> Demux2/1
  Mux2/1 -> VR_cord/1
  Demux2/3 -> Mux2/2
  Demux2/1 -> Mux2/3
  Demux2/2 -> Mux2/1

== system observerModel_GVS/Quaternion Rotator/Quaternion Integrator/delta_q ==
  omega : Inport
  q : Inport  Port=2
  C : Subsystem
  Constant : Constant  Value=delta_t
  K : Subsystem
  Product : Product  RndMeth=Zero
  Product1 : Product  RndMeth=Zero
  Product2 : Product  RndMeth=Zero
  Sum : Sum
  Z : Subsystem
  delta_q : Outport
  wires:
  q/1 -> C/2(q), Z/1(q), Product1/1
  Z/1(z) -> Product/1
  Product/1 -> Product1/2
  Product1/1 -> Sum/2
  C/1(C) -> Sum/1
  Sum/1 -> Product2/2
  Constant/1 -> Product2/1
  omega/1 -> C/1(omega)
  Product2/1 -> delta_q/1
  K/1(K) -> Product/2

== system observerModel_GVS/Quaternion Rotator/Quaternion to Direction Cosine/A1 ==
  q : Inport
  Demux : Demux
  Gain : Gain  Gain=2
  Product : Product  RndMeth=Zero
  Product1 : Product  RndMeth=Zero
  Sum : Sum  Inputs=+-
  A21 : Outport
  wires:
  q/1 -> Demux/1
  Sum/1 -> Gain/1
  Gain/1 -> A21/1
  Product/1 -> Sum/1
  Product1/1 -> Sum/2
  Demux/2 -> Product/1
  Demux/3 -> Product/2
  Demux/1 -> Product1/1
  Demux/4 -> Product1/2

== system observerModel_GVS/Quaternion Rotator/Quaternion to Direction Cosine/A11 ==
  q : Inport
  Demux : Demux
  Product{,1..3} (4 alike) : Product  RndMeth=Zero
  Sum : Sum  Inputs=++--
  A11 : Outport
  wires:
  Demux/1 -> Product/1, Product/2
  Demux/2 -> Product1/1, Product1/2
  Demux/3 -> Product2/1, Product2/2
  Demux/4 -> Product3/1, Product3/2
  Product/1 -> Sum/1
  Product1/1 -> Sum/2
  Product2/1 -> Sum/3
  Product3/1 -> Sum/4
  q/1 -> Demux/1
  Sum/1 -> A11/1

== system observerModel_GVS/Quaternion Rotator/Quaternion to Direction Cosine/A12 ==
  q : Inport
  Demux : Demux
  Gain : Gain  Gain=2
  Product : Product  RndMeth=Zero
  Product1 : Product  RndMeth=Zero
  Sum : Sum
  A12 : Outport
  wires:
  q/1 -> Demux/1
  Sum/1 -> Gain/1
  Gain/1 -> A12/1
  Demux/2 -> Product/1
  Demux/3 -> Product/2
  Demux/1 -> Product1/1
  Demux/4 -> Product1/2
  Product/1 -> Sum/1
  Product1/1 -> Sum/2

== system observerModel_GVS/Quaternion Rotator/Quaternion to Direction Cosine/A13 ==
  q : Inport
  Demux : Demux
  Gain : Gain  Gain=2
  Product : Product  RndMeth=Zero
  Product1 : Product  RndMeth=Zero
  Sum : Sum  Inputs=+-
  A13 : Outport
  wires:
  q/1 -> Demux/1
  Sum/1 -> Gain/1
  Gain/1 -> A13/1
  Product/1 -> Sum/1
  Product1/1 -> Sum/2
  Demux/2 -> Product/1
  Demux/4 -> Product/2
  Demux/1 -> Product1/1
  Demux/3 -> Product1/2

== system observerModel_GVS/Quaternion Rotator/Quaternion to Direction Cosine/A22 ==
  q : Inport
  Demux : Demux
  Product{,1..3} (4 alike) : Product  RndMeth=Zero
  Sum : Sum  Inputs=+-+-
  A22 : Outport
  wires:
  Demux/1 -> Product/1, Product/2
  Demux/2 -> Product1/1, Product1/2
  Demux/3 -> Product2/1, Product2/2
  Demux/4 -> Product3/1, Product3/2
  Product/1 -> Sum/1
  Product1/1 -> Sum/2
  Product2/1 -> Sum/3
  Product3/1 -> Sum/4
  q/1 -> Demux/1
  Sum/1 -> A22/1

== system observerModel_GVS/Quaternion Rotator/Quaternion to Direction Cosine/A23 ==
  q : Inport
  Demux : Demux
  Gain : Gain  Gain=2
  Product : Product  RndMeth=Zero
  Product1 : Product  RndMeth=Zero
  Sum : Sum
  A23 : Outport
  wires:
  q/1 -> Demux/1
  Sum/1 -> Gain/1
  Gain/1 -> A23/1
  Product/1 -> Sum/1
  Product1/1 -> Sum/2
  Demux/3 -> Product1/1
  Demux/4 -> Product1/2
  Demux/1 -> Product/1
  Demux/2 -> Product/2

== system observerModel_GVS/Quaternion Rotator/Quaternion to Direction Cosine/A31 ==
  q : Inport
  Demux : Demux
  Gain : Gain  Gain=2
  Product : Product  RndMeth=Zero
  Product1 : Product  RndMeth=Zero
  Sum : Sum
  A31 : Outport
  wires:
  q/1 -> Demux/1
  Sum/1 -> Gain/1
  Gain/1 -> A31/1
  Product/1 -> Sum/1
  Product1/1 -> Sum/2
  Demux/1 -> Product/1
  Demux/3 -> Product/2
  Demux/2 -> Product1/1
  Demux/4 -> Product1/2

== system observerModel_GVS/Quaternion Rotator/Quaternion to Direction Cosine/A32 ==
  q : Inport
  Demux : Demux
  Gain : Gain  Gain=2
  Product : Product  RndMeth=Zero
  Product1 : Product  RndMeth=Zero
  Sum : Sum  Inputs=+-
  A32 : Outport
  wires:
  q/1 -> Demux/1
  Sum/1 -> Gain/1
  Gain/1 -> A32/1
  Product/1 -> Sum/1
  Product1/1 -> Sum/2
  Demux/3 -> Product/1
  Demux/4 -> Product/2
  Demux/1 -> Product1/1
  Demux/2 -> Product1/2

== system observerModel_GVS/Quaternion Rotator/Quaternion to Direction Cosine/A33 ==
  q : Inport
  Demux : Demux
  Product{,1..3} (4 alike) : Product  RndMeth=Zero
  Sum : Sum  Inputs=+--+
  A33 : Outport
  wires:
  Demux/1 -> Product/1, Product/2
  Demux/2 -> Product1/1, Product1/2
  Demux/3 -> Product2/1, Product2/2
  Demux/4 -> Product3/1, Product3/2
  Product/1 -> Sum/1
  Product1/1 -> Sum/2
  Product2/1 -> Sum/3
  Product3/1 -> Sum/4
  q/1 -> Demux/1
  Sum/1 -> A33/1

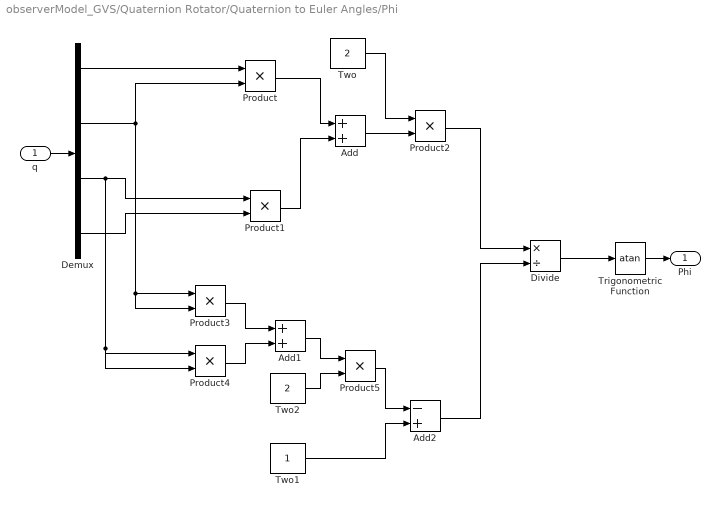
== system observerModel_GVS/Quaternion Rotator/Quaternion to Euler Angles/Phi ==
  q : Inport
  Add : Sum
  Add1 : Sum
  Add2 : Sum  Inputs=-+
  Demux : Demux
  Divide : Product  Inputs=*/
  Product{,1..5} (6 alike) : Product  RndMeth=Zero
  Trigonometric Function : Trigonometry  Operator=atan
  Two : Constant  Value=2  VectorParams1D=off
  Two1 : Constant  VectorParams1D=off
  Two2 : Constant  Value=2  VectorParams1D=off
  Phi : Outport
  wires:
  Demux/1 -> Product/1
  Demux/2 -> Product/2, Product3/1, Product3/2
  Product/1 -> Add/1
  Demux/4 -> Product1/2
  Demux/3 -> Product1/1, Product4/1, Product4/2
  Product1/1 -> Add/2
  Add/1 -> Product2/2
  Two/1 -> Product2/1
  Product3/1 -> Add1/1
  Product4/1 -> Add1/2
  Add1/1 -> Product5/1
  Two2/1 -> Product5/2
  Product5/1 -> Add2/1
  Two1/1 -> Add2/2
  Product2/1 -> Divide/1
  Add2/1 -> Divide/2
  Divide/1 -> Trigonometric Function/1
  q/1 -> Demux/1
  Trigonometric Function/1 -> Phi/1

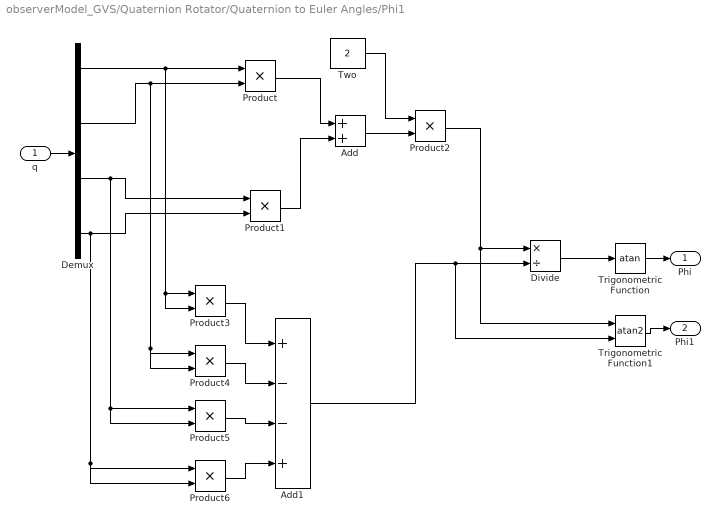
== system observerModel_GVS/Quaternion Rotator/Quaternion to Euler Angles/Phi1 ==
  q : Inport
  Add : Sum
  Add1 : Sum  Inputs=+--+
  Demux : Demux
  Divide : Product  Inputs=*/
  Product{,1..6} (7 alike) : Product  RndMeth=Zero
  Trigonometric Function : Trigonometry  Operator=atan
  Trigonometric Function1 : Trigonometry  Operator=atan2
  Two : Constant  Value=2  VectorParams1D=off
  Phi : Outport
  Phi1 : Outport  Port=2
  wires:
  Demux/1 -> Product/1, Product3/1, Product3/2
  Demux/2 -> Product/2, Product4/1, Product4/2
  Product/1 -> Add/1
  Demux/4 -> Product1/2, Product6/1, Product6/2
  Demux/3 -> Product1/1, Product5/1, Product5/2
  Product1/1 -> Add/2
  Add/1 -> Product2/2
  Two/1 -> Product2/1
  Product3/1 -> Add1/1
  Product4/1 -> Add1/2
  Product2/1 -> Divide/1, Trigonometric Function1/1
  Divide/1 -> Trigonometric Function/1
  q/1 -> Demux/1
  Trigonometric Function/1 -> Phi/1
  Product5/1 -> Add1/3
  Product6/1 -> Add1/4
  Add1/1 -> Divide/2, Trigonometric Function1/2
  Trigonometric Function1/1 -> Phi1/1

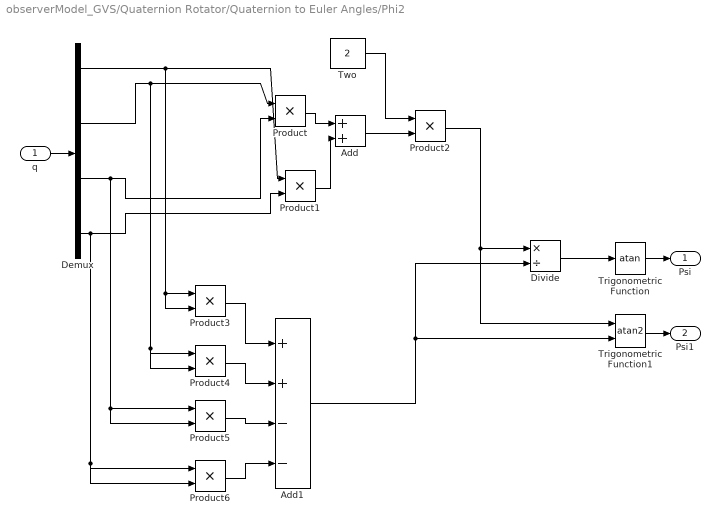
== system observerModel_GVS/Quaternion Rotator/Quaternion to Euler Angles/Phi2 ==
  q : Inport
  Add : Sum
  Add1 : Sum  Inputs=++--
  Demux : Demux
  Divide : Product  Inputs=*/
  Product{,1..6} (7 alike) : Product  RndMeth=Zero
  Trigonometric Function : Trigonometry  Operator=atan
  Trigonometric Function1 : Trigonometry  Operator=atan2
  Two : Constant  Value=2  VectorParams1D=off
  Psi : Outport
  Psi1 : Outport  Port=2
  wires:
  Demux/1 -> Product3/1, Product3/2, Product1/1
  Demux/2 -> Product4/1, Product4/2, Product/1
  Demux/4 -> Product6/1, Product6/2, Product1/2
  Demux/3 -> Product5/1, Product5/2, Product/2
  Add/1 -> Product2/2
  Two/1 -> Product2/1
  Product3/1 -> Add1/1
  Product4/1 -> Add1/2
  Product2/1 -> Divide/1, Trigonometric Function1/1
  Divide/1 -> Trigonometric Function/1
  q/1 -> Demux/1
  Trigonometric Function/1 -> Psi/1
  Product5/1 -> Add1/3
  Product6/1 -> Add1/4
  Add1/1 -> Divide/2, Trigonometric Function1/2
  Product1/1 -> Add/2
  Product/1 -> Add/1
  Trigonometric Function1/1 -> Psi1/1

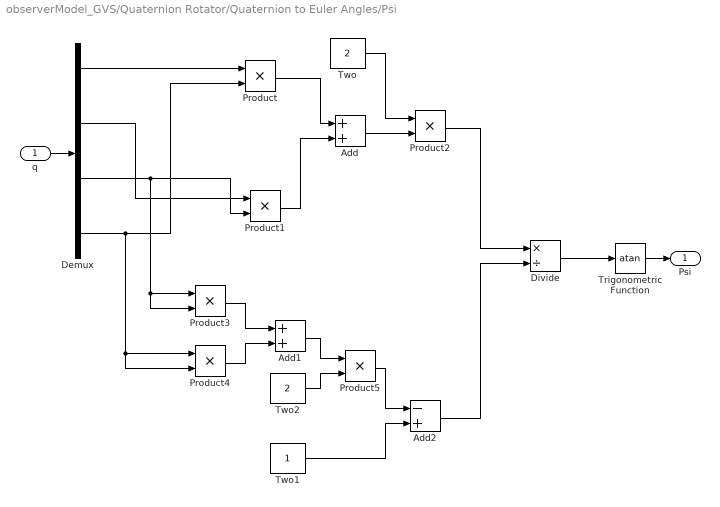
== system observerModel_GVS/Quaternion Rotator/Quaternion to Euler Angles/Psi ==
  q : Inport
  Add : Sum
  Add1 : Sum
  Add2 : Sum  Inputs=-+
  Demux : Demux
  Divide : Product  Inputs=*/
  Product{,1..5} (6 alike) : Product  RndMeth=Zero
  Trigonometric Function : Trigonometry  Operator=atan
  Two : Constant  Value=2  VectorParams1D=off
  Two1 : Constant  VectorParams1D=off
  Two2 : Constant  Value=2  VectorParams1D=off
  Psi : Outport
  wires:
  Demux/2 -> Product1/1
  Product/1 -> Add/1
  Demux/4 -> Product4/1, Product4/2, Product/2
  Product1/1 -> Add/2
  Add/1 -> Product2/2
  Two/1 -> Product2/1
  Product3/1 -> Add1/1
  Product4/1 -> Add1/2
  Add1/1 -> Product5/1
  Two2/1 -> Product5/2
  Product5/1 -> Add2/1
  Two1/1 -> Add2/2
  Product2/1 -> Divide/1
  Add2/1 -> Divide/2
  Divide/1 -> Trigonometric Function/1
  q/1 -> Demux/1
  Trigonometric Function/1 -> Psi/1
  Demux/1 -> Product/1
  Demux/3 -> Product1/2, Product3/1, Product3/2

== system observerModel_GVS/Quaternion Rotator/Quaternion to Euler Angles/Theta ==
  q : Inport
  Add : Sum  Inputs=+-
  Demux : Demux
  Product : Product  RndMeth=Zero
  Product1 : Product  RndMeth=Zero
  Product2 : Product  RndMeth=Zero
  Trigonometric Function : Trigonometry  Operator=asin
  Two : Constant  Value=2  VectorParams1D=off
  Theta : Outport
  wires:
  Demux/1 -> Product/1
  Product/1 -> Add/1
  Demux/4 -> Product1/2
  Product1/1 -> Add/2
  Add/1 -> Product2/2
  Two/1 -> Product2/1
  q/1 -> Demux/1
  Trigonometric Function/1 -> Theta/1
  Product2/1 -> Trigonometric Function/1
  Demux/3 -> Product/2
  Demux/2 -> Product1/1

== system observerModel_GVS/Quaternion Rotator/Quaternion to Euler Angles/Theta1 ==
  q : Inport
  Add : Sum  Inputs=+-
  Demux : Demux
  Product : Product  RndMeth=Zero
  Product1 : Product  RndMeth=Zero
  Product2 : Product  RndMeth=Zero
  Trigonometric Function : Trigonometry  Operator=asin
  Two : Constant  Value=2  VectorParams1D=off
  Theta : Outport
  wires:
  Demux/1 -> Product/1
  Product/1 -> Add/1
  Demux/4 -> Product1/2
  Product1/1 -> Add/2
  Add/1 -> Product2/2
  Two/1 -> Product2/1
  q/1 -> Demux/1
  Trigonometric Function/1 -> Theta/1
  Product2/1 -> Trigonometric Function/1
  Demux/3 -> Product/2
  Demux/2 -> Product1/1

== system observerModel_GVS/Quaternion Rotator/Rotation/Azimuthal Integrator ==
  g : Inport
  D_Cos : Inport  Port=2
  omega_rad : Inport  Port=3
  Dot Product : DotProduct  OutDataTypeStr=Inherit: Inherit via internal rule
  Gain : Gain  Gain=180/3.14159
  Integrator : Integrator
  Matrix Multiplication1 : Subsystem
  Scope1 : Scope
  azimuth : Outport
  wires:
  Matrix Multiplication1/1(omega_rad') -> Dot Product/2
  Dot Product/1 -> Gain/1, Integrator/1
  Gain/1 -> Scope1/1
  Integrator/1 -> azimuth/1
  g/1 -> Dot Product/1
  D_Cos/1 -> Matrix Multiplication1/1(D_Cos)
  omega_rad/1 -> Matrix Multiplication1/2(omega_rad)

== system observerModel_GVS/Quaternion Rotator/Rotation/Matrix Multiplication ==
  D_Cos : Inport
  G0 : Inport  Port=2
  Demux : Demux  Outputs=3
      settings: DisplayOption=none
  Mux : Mux  Inputs=3
  Product : Product  Multiplication=Matrix(*)  RndMeth=Zero
  g : Outport
  wires:
  Product/1 -> Demux/1
  Demux/1 -> Mux/1
  Demux/2 -> Mux/2
  Demux/3 -> Mux/3
  D_Cos/1 -> Product/1
  Mux/1 -> g/1
  G0/1 -> Product/2

== system observerModel_GVS/Quaternion Rotator/Tilt & SVV/SVV Calculator ==
  g : Inport
  Demux : Demux  Outputs=3
  Divide : Product  Inputs=*/
  Terminator : Terminator
  Trigonometric Function : Trigonometry  Operator=atan
  SVV : Outport
  wires:
  Divide/1 -> Trigonometric Function/1
  g/1 -> Demux/1
  Trigonometric Function/1 -> SVV/1
  Demux/2 -> Divide/1
  Demux/3 -> Divide/2
  Demux/1 -> Terminator/1

== system observerModel_GVS/Quaternion Rotator/Tilt & SVV/Tilt Calculator ==
  g : Inport
  Add : Sum  Inputs=+++
  Demux : Demux  Outputs=3
  Divide : Product  Inputs=*/
  Math Function : Math  Operator=sqrt  SignedPower=on
  Product{,1..3} (4 alike) : Product  RndMeth=Zero
  Trigonometric Function : Trigonometry  Operator=acos  OutputSignalType=real
  Two : Constant  Value=-1  VectorParams1D=off
  Tilt : Outport
  wires:
  Product/1 -> Add/1
  Product1/1 -> Add/2
  Divide/1 -> Trigonometric Function/1
  g/1 -> Demux/1
  Product2/1 -> Add/3
  Demux/1 -> Product/1, Product/2
  Demux/2 -> Product1/2, Product1/1
  Demux/3 -> Product2/2, Product2/1, Product3/1
  Add/1 -> Math Function/1
  Two/1 -> Product3/2
  Math Function/1 -> Divide/2
  Product3/1 -> Divide/1
  Trigonometric Function/1 -> Tilt/1
